simulink model "TankAController"  (Simulink 8.1)
settings: Solver=ode45  StartTime=0.0  StopTime=10.0  RelTol=1e-3
settings Model: Creator=root  LastModifiedBy=root
settings DataIOCC: SignalLoggingSaveFormat=Dataset
settings OptimizationCC: ExpressionDepthLimit=128
settings DebuggingCC: FcnCallInpInsideContextMsg=EnableAllAsError
settings GRTTargetCC: CombineOutputUpdateFcns=on  GRTInterface=off

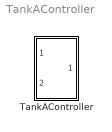
== system TankAController ==
  TankAController : Subsystem

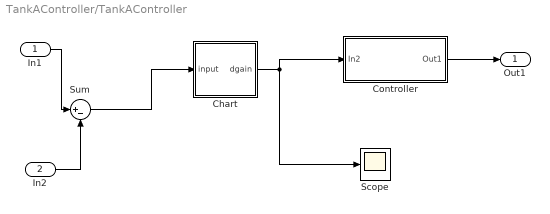
== system TankAController/TankAController ==
  In1 : Inport  OutDataTypeStr=double
  In2 : Inport  Port=2  OutDataTypeStr=double
  Chart : Stateflow chart  TreatAsAtomicUnit=on
  Controller : Subsystem
  Scope : Scope
      settings: SaveName=ScopeData2
  Sum : Sum  Inputs=|+-
  Out1 : Outport  OutDataTypeStr=double
  wires:
  Controller/1(Out1) -> Out1/1
  In1/1 -> Sum/1
  Chart/1(dgain) -> Scope/1, Controller/1(In2)
  Sum/1 -> Chart/1(input)
  In2/1 -> Sum/2

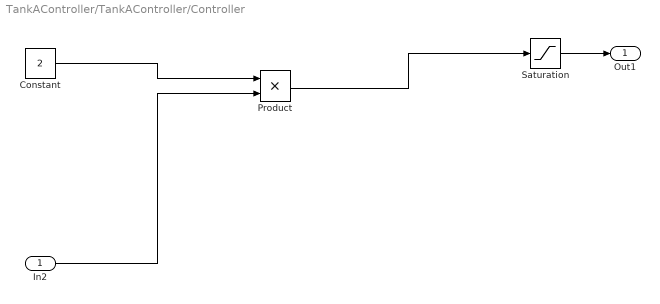
== system TankAController/TankAController/Controller ==
  In2 : Inport
  Constant : Constant  Value=2
  Product : Product
  Saturation : Saturate  UpperLimit=10  LowerLimit=0
  Out1 : Outport
  wires:
  Saturation/1 -> Out1/1
  In2/1 -> Product/2
  Product/1 -> Saturation/1
  Constant/1 -> Product/1

== stateflow chart TankAController/Chart ==
  state High
    entry: dgain = 1
  state Medium
    entry: dgain = 0.5
  state Off
    entry: dgain = 0
  (default) -> High
  Medium -> High [order 1] : [input > 2]
  High -> Medium : [input < 2]
  Off -> Medium : [input > 2]
  Medium -> Off [order 2] : [input < 0]
  data: input input double; dgain output double
